simulink model "EngineModel_scaled_15_7_2016_with_new_maps"  (R2021a)
settings: Solver=ode4  StartTime=0.0  StopTime=30  FixedStep=0.2  RelTol=1e-3  EnableMultiTasking=on
values from neighbouring files (symbols this model uses):
  Fanmap_2 = [1 1 1 1 1 1 1 1 1 1 275.724 325.4224 ... (330 elements, 10x3x11)]    [enginemaps2.mat]
  HPCompmap_2 = [1 1 1 1 1 1 1 1 1 1 32.390865 37.6623195 ... (330 elements, 10x3x11)]    [enginemaps2.mat]
  HPTurbinemap_2 = [0.24979968 0.24979968 0.24979968 0.24979968 0.24979968 0.24979968 0.24979968 0.24979968 0.24979968 0.24979968 0.004250667 0.005047667 ... (330 elements, 10x3x11)]    [enginemaps2.mat]
  LPCompmap_2 = [1 1 1 1 1 1 1 1 1 1 34.17260994 40.23277722 ... (330 elements, 10x3x11)]    [enginemaps2.mat]
  LPTurbinemap_2 = [0.665969797 0.665969797 0.665969797 0.665969797 0.665969797 0.665969797 0.665969797 0.665969797 0.00912 0.013173333 0.015706667 0.01672 ... (264 elements, 8x3x11)]    [enginemaps2.mat]
undefined symbols (not defined in the file or in its folder): Adiabatic_compression_fan, Adiabatic_compression_HPC, Adiabatic_compression_LPC, coldnozzle, compression_ram, cond_f2, D, datatables, hotnozzle, HPT1, if_Nth, if_Ntl, if_Z, LPT, performance1, thermo_combustor, turbo
libraries: dspmtrx3 x10, aerolibatmos2 x8, dspsigattribs x3, dspsolvers x2, dspfactors x1
(part 13 of 13)

== system EngineModel_scaled_15_7_2016_with_new_maps/Double spool TFE CF6-50 steady state modeling (BOING 747-200)/Error Due to Vs/Error Due To Dv6/LPT/enthalpy_MAPS/LPT map/LPT Map lookup Table (DH//T) ==
  corr speed Ntl : Inport
  TFtl : Inport  Port=2
  3D LPTurbinemap Lookup Table (DH/T) : Lookup_n-D  NumberOfTableDimensions=3  BreakpointsForDimension1=[461.059151,535.7395809,608.9086832,673.9999999,735.0784813,781.7211783,815.12673,850.3562978]  BreakpointsForDimension2=[1,2,3]  BreakpointsForDimension3=[0,0.1,0.2,0.3,0.4,0.5,0.6,0.7,0.8,0.9,1]  IndexSearchMethod=Linear search  Table=LPTurbinemap_2  InterpMethod=Cubic spline  ExtrapMethod=Cubic spline  OutDataTypeStr=double  RndMeth=Simplest
      settings: InputPortMap=u0,u1,u2
  Constant1 : Constant  Value=2
  Display : Display
  If condition Ztl : Subsystem
  if_Ntl : Subsystem
  LPT (DH/T)tl : Outport
  wires:
  corr speed Ntl/1 -> if_Ntl/2(Ntl)
  if_Ntl/1(Ztli) -> If condition Ztl/1(Ztli)
  If condition Ztl/1(Ztl) -> 3D LPTurbinemap Lookup Table (DH/T)/3
  TFtl/1 -> 3D LPTurbinemap Lookup Table (DH/T)/1, if_Ntl/1(TFtl)
  Constant1/1 -> 3D LPTurbinemap Lookup Table (DH/T)/2
  3D LPTurbinemap Lookup Table (DH/T)/1 -> Display/1, LPT (DH/T)tl/1

== system EngineModel_scaled_15_7_2016_with_new_maps/Double spool TFE CF6-50 steady state modeling (BOING 747-200)/Error Due to Vs/Error Due To Dv6/LPT/enthalpy_MAPS/LPT map/LPT Map lookup Table Efficency ==
  corr speed Ntl : Inport
  TFtl : Inport  Port=2
  3D LPTurbinemap Lookup Table Effienicy : Lookup_n-D  NumberOfTableDimensions=3  BreakpointsForDimension1=[461.059151,535.7395809,608.9086832,673.9999999,735.0784813,781.7211783,815.12673,850.3562978]  BreakpointsForDimension2=[1,2,3]  BreakpointsForDimension3=[0,0.1,0.2,0.3,0.4,0.5,0.6,0.7,0.8,0.9,1]  IndexSearchMethod=Linear search  Table=LPTurbinemap_2  InterpMethod=Cubic spline  ExtrapMethod=Cubic spline  OutDataTypeStr=double  RndMeth=Simplest
      settings: InputPortMap=u0,u1,u2
  Constant1 : Constant  Value=3
  Display : Display
  If condition Ztl : Subsystem
  if_Ntl : Subsystem
  HPT Ettatl : Outport
  wires:
  corr speed Ntl/1 -> if_Ntl/2(Ntl)
  if_Ntl/1(Ztli) -> If condition Ztl/1(Ztli)
  If condition Ztl/1(Ztl) -> 3D LPTurbinemap Lookup Table Effienicy/3
  TFtl/1 -> 3D LPTurbinemap Lookup Table Effienicy/1, if_Ntl/1(TFtl)
  Constant1/1 -> 3D LPTurbinemap Lookup Table Effienicy/2
  3D LPTurbinemap Lookup Table Effienicy/1 -> Display/1, HPT Ettatl/1

== system EngineModel_scaled_15_7_2016_with_new_maps/Double spool TFE CF6-50 steady state modeling (BOING 747-200)/Error Due to Vs/Error Due To Dv7/HPT/enthalpy_MAPS/HPT map/HPT Map lookup Table (DH//T) ==
  corr speed Nth : Inport
  TFth : Inport  Port=2
  3D HPTurbinemap Lookup Table (DH/T) : Lookup_n-D  NumberOfTableDimensions=3  BreakpointsForDimension1=[124.08776,134.47272,148.45488,152.05208,153.8194,155.1488,156.4,157.7294,159.27776,161.3266]  BreakpointsForDimension2=[1,2,3]  BreakpointsForDimension3=[0,0.1,0.2,0.3,0.4,0.5,0.6,0.7,0.8,0.9,1]  IndexSearchMethod=Linear search  Table=HPTurbinemap_2  InterpMethod=Cubic spline  ExtrapMethod=Cubic spline  OutDataTypeStr=double  RndMeth=Simplest
      settings: InputPortMap=u0,u1,u2
  Constant1 : Constant  Value=2
  Display : Display
  If condition Zth : Subsystem
  if_Nth : Subsystem
  HPT (DH/T)th : Outport
  wires:
  3D HPTurbinemap Lookup Table (DH/T)/1 -> HPT (DH/T)th/1, Display/1
  TFth/1 -> if_Nth/1(TFth), 3D HPTurbinemap Lookup Table (DH/T)/1
  Constant1/1 -> 3D HPTurbinemap Lookup Table (DH/T)/2
  If condition Zth/1(Zth) -> 3D HPTurbinemap Lookup Table (DH/T)/3
  if_Nth/1(Zthi) -> If condition Zth/1(Zthi)
  corr speed Nth/1 -> if_Nth/2(Nth)

== system EngineModel_scaled_15_7_2016_with_new_maps/Double spool TFE CF6-50 steady state modeling (BOING 747-200)/Error Due to Vs/Error Due To Dv7/HPT/enthalpy_MAPS/HPT map/HPT Map lookup Table Efficency ==
  corr speed Nth : Inport
  TFth : Inport  Port=2
  3D HPTurbinemap Lookup Table Efficency : Lookup_n-D  NumberOfTableDimensions=3  BreakpointsForDimension1=[124.08776,134.47272,148.45488,152.05208,153.8194,155.1488,156.4,157.7294,159.27776,161.3266]  BreakpointsForDimension2=[1,2,3]  BreakpointsForDimension3=[0,0.1,0.2,0.3,0.4,0.5,0.6,0.7,0.8,0.9,1]  IndexSearchMethod=Linear search  Table=HPTurbinemap_2  InterpMethod=Cubic spline  ExtrapMethod=Cubic spline  OutDataTypeStr=double  RndMeth=Simplest
      settings: InputPortMap=u0,u1,u2
  Constant1 : Constant  Value=3
  Display : Display
  Display1 : Display
  If condition Zf : Subsystem
  if_Nth : Subsystem
  HPT Ettath : Outport
  wires:
  3D HPTurbinemap Lookup Table Efficency/1 -> HPT Ettath/1, Display/1
  Constant1/1 -> 3D HPTurbinemap Lookup Table Efficency/2
  TFth/1 -> if_Nth/1(TFth), 3D HPTurbinemap Lookup Table Efficency/1
  if_Nth/1(Zthi) -> If condition Zf/1(Zthi)
  corr speed Nth/1 -> if_Nth/2(Nth)
  If condition Zf/1(Zth) -> Display1/1, 3D HPTurbinemap Lookup Table Efficency/3

== system EngineModel_scaled_15_7_2016_with_new_maps/Double spool TFE CF6-50 steady state modeling (BOING 747-200)/Error Due to Vs/Error Due To Dv7/LPT/enthalpy_MAPS/LPT map/LPT Map lookup Table (DH//T) ==
  corr speed Ntl : Inport
  TFtl : Inport  Port=2
  3D LPTurbinemap Lookup Table (DH/T) : Lookup_n-D  NumberOfTableDimensions=3  BreakpointsForDimension1=[461.059151,535.7395809,608.9086832,673.9999999,735.0784813,781.7211783,815.12673,850.3562978]  BreakpointsForDimension2=[1,2,3]  BreakpointsForDimension3=[0,0.1,0.2,0.3,0.4,0.5,0.6,0.7,0.8,0.9,1]  IndexSearchMethod=Linear search  Table=LPTurbinemap_2  InterpMethod=Cubic spline  ExtrapMethod=Cubic spline  OutDataTypeStr=double  RndMeth=Simplest
      settings: InputPortMap=u0,u1,u2
  Constant1 : Constant  Value=2
  Display : Display
  If condition Ztl : Subsystem
  if_Ntl : Subsystem
  LPT (DH/T)tl : Outport
  wires:
  3D LPTurbinemap Lookup Table (DH/T)/1 -> LPT (DH/T)tl/1, Display/1
  Constant1/1 -> 3D LPTurbinemap Lookup Table (DH/T)/2
  TFtl/1 -> if_Ntl/1(TFtl), 3D LPTurbinemap Lookup Table (DH/T)/1
  If condition Ztl/1(Ztl) -> 3D LPTurbinemap Lookup Table (DH/T)/3
  if_Ntl/1(Ztli) -> If condition Ztl/1(Ztli)
  corr speed Ntl/1 -> if_Ntl/2(Ntl)

== system EngineModel_scaled_15_7_2016_with_new_maps/Double spool TFE CF6-50 steady state modeling (BOING 747-200)/Error Due to Vs/Error Due To Dv7/LPT/enthalpy_MAPS/LPT map/LPT Map lookup Table Efficency ==
  corr speed Ntl : Inport
  TFtl : Inport  Port=2
  3D LPTurbinemap Lookup Table Effienicy : Lookup_n-D  NumberOfTableDimensions=3  BreakpointsForDimension1=[461.059151,535.7395809,608.9086832,673.9999999,735.0784813,781.7211783,815.12673,850.3562978]  BreakpointsForDimension2=[1,2,3]  BreakpointsForDimension3=[0,0.1,0.2,0.3,0.4,0.5,0.6,0.7,0.8,0.9,1]  IndexSearchMethod=Linear search  Table=LPTurbinemap_2  InterpMethod=Cubic spline  ExtrapMethod=Cubic spline  OutDataTypeStr=double  RndMeth=Simplest
      settings: InputPortMap=u0,u1,u2
  Constant1 : Constant  Value=3
  Display : Display
  If condition Ztl : Subsystem
  if_Ntl : Subsystem
  HPT Ettatl : Outport
  wires:
  3D LPTurbinemap Lookup Table Effienicy/1 -> HPT Ettatl/1, Display/1
  Constant1/1 -> 3D LPTurbinemap Lookup Table Effienicy/2
  TFtl/1 -> if_Ntl/1(TFtl), 3D LPTurbinemap Lookup Table Effienicy/1
  If condition Ztl/1(Ztl) -> 3D LPTurbinemap Lookup Table Effienicy/3
  if_Ntl/1(Ztli) -> If condition Ztl/1(Ztli)
  corr speed Ntl/1 -> if_Ntl/2(Ntl)

== system EngineModel_scaled_15_7_2016_with_new_maps/Double spool TFE CF6-50 steady state modeling (BOING 747-200)/Off- Design Module/HPT/enthalpy_MAPS/HPT map/HPT Map lookup Table (DH//T)/If condition Zth ==
  Zthi : Inport
  Demux : Demux  Outputs=1
      settings: DisplayOption=none
  Interpreted MATLAB Function : MATLABFcn  MATLABFcn=if_Z(u(1))  OutputDimensions=1
  Mux : Mux  Inputs=1
      settings: DisplayOption=signals
  Zth : Outport
  wires:
  Interpreted MATLAB Function/1 -> Demux/1
  Mux/1 -> Interpreted MATLAB Function/1
  Demux/1 -> Zth/1
  Zthi/1 -> Mux/1

== system EngineModel_scaled_15_7_2016_with_new_maps/Double spool TFE CF6-50 steady state modeling (BOING 747-200)/Off- Design Module/HPT/enthalpy_MAPS/HPT map/HPT Map lookup Table (DH//T)/if_Nth ==
  TFth : Inport
  Nth : Inport  Port=2
  Demux : Demux  Outputs=1
      settings: DisplayOption=none
  Interpreted MATLAB Function : MATLABFcn  MATLABFcn=if_Nth(u(1),u(2))  OutputDimensions=1
  Mux : Mux  Inputs=2
      settings: DisplayOption=signals
  Zthi : Outport
  wires:
  Interpreted MATLAB Function/1 -> Demux/1
  TFth/1 -> Mux/1
  Mux/1 -> Interpreted MATLAB Function/1
  Demux/1 -> Zthi/1
  Nth/1 -> Mux/2

== system EngineModel_scaled_15_7_2016_with_new_maps/Double spool TFE CF6-50 steady state modeling (BOING 747-200)/Off- Design Module/HPT/enthalpy_MAPS/HPT map/HPT Map lookup Table Efficency/If condition Zf ==
  Zthi : Inport
  Demux : Demux  Outputs=1
      settings: DisplayOption=none
  Interpreted MATLAB Function : MATLABFcn  MATLABFcn=if_Z(u(1))  OutputDimensions=1
  Mux : Mux  Inputs=1
      settings: DisplayOption=signals
  Zth : Outport
  wires:
  Interpreted MATLAB Function/1 -> Demux/1
  Mux/1 -> Interpreted MATLAB Function/1
  Demux/1 -> Zth/1
  Zthi/1 -> Mux/1

== system EngineModel_scaled_15_7_2016_with_new_maps/Double spool TFE CF6-50 steady state modeling (BOING 747-200)/Off- Design Module/HPT/enthalpy_MAPS/HPT map/HPT Map lookup Table Efficency/if_Nth ==
  TFth : Inport
  Nth : Inport  Port=2
  Demux : Demux  Outputs=1
      settings: DisplayOption=none
  Interpreted MATLAB Function : MATLABFcn  MATLABFcn=if_Nth(u(1),u(2))  OutputDimensions=1
  Mux : Mux  Inputs=2
      settings: DisplayOption=signals
  Zthi : Outport
  wires:
  Interpreted MATLAB Function/1 -> Demux/1
  TFth/1 -> Mux/1
  Mux/1 -> Interpreted MATLAB Function/1
  Demux/1 -> Zthi/1
  Nth/1 -> Mux/2

== system EngineModel_scaled_15_7_2016_with_new_maps/Double spool TFE CF6-50 steady state modeling (BOING 747-200)/Off- Design Module/LPT/enthalpy_MAPS/LPT map/LPT Map lookup Table (DH//T)/If condition Ztl ==
  Ztli : Inport
  Demux : Demux  Outputs=1
      settings: DisplayOption=none
  Interpreted MATLAB Function : MATLABFcn  MATLABFcn=if_Z(u(1))  OutputDimensions=1
  Mux : Mux  Inputs=1
      settings: DisplayOption=signals
  Ztl : Outport
  wires:
  Interpreted MATLAB Function/1 -> Demux/1
  Mux/1 -> Interpreted MATLAB Function/1
  Demux/1 -> Ztl/1
  Ztli/1 -> Mux/1

== system EngineModel_scaled_15_7_2016_with_new_maps/Double spool TFE CF6-50 steady state modeling (BOING 747-200)/Off- Design Module/LPT/enthalpy_MAPS/LPT map/LPT Map lookup Table (DH//T)/if_Ntl ==
  TFtl : Inport
  Ntl : Inport  Port=2
  Demux : Demux  Outputs=1
      settings: DisplayOption=none
  Interpreted MATLAB Function : MATLABFcn  MATLABFcn=if_Ntl(u(1),u(2))  OutputDimensions=1
  Mux : Mux  Inputs=2
      settings: DisplayOption=signals
  Ztli : Outport
  wires:
  Interpreted MATLAB Function/1 -> Demux/1
  TFtl/1 -> Mux/1
  Mux/1 -> Interpreted MATLAB Function/1
  Demux/1 -> Ztli/1
  Ntl/1 -> Mux/2

== system EngineModel_scaled_15_7_2016_with_new_maps/Double spool TFE CF6-50 steady state modeling (BOING 747-200)/Off- Design Module/LPT/enthalpy_MAPS/LPT map/LPT Map lookup Table Efficency/If condition Ztl ==
  Ztli : Inport
  Demux : Demux  Outputs=1
      settings: DisplayOption=none
  Interpreted MATLAB Function : MATLABFcn  MATLABFcn=if_Z(u(1))  OutputDimensions=1
  Mux : Mux  Inputs=1
      settings: DisplayOption=signals
  Ztl : Outport
  wires:
  Interpreted MATLAB Function/1 -> Demux/1
  Mux/1 -> Interpreted MATLAB Function/1
  Demux/1 -> Ztl/1
  Ztli/1 -> Mux/1

== system EngineModel_scaled_15_7_2016_with_new_maps/Double spool TFE CF6-50 steady state modeling (BOING 747-200)/Off- Design Module/LPT/enthalpy_MAPS/LPT map/LPT Map lookup Table Efficency/if_Ntl ==
  TFtl : Inport
  Ntl : Inport  Port=2
  Demux : Demux  Outputs=1
      settings: DisplayOption=none
  Interpreted MATLAB Function : MATLABFcn  MATLABFcn=if_Ntl(u(1),u(2))  OutputDimensions=1
  Mux : Mux  Inputs=2
      settings: DisplayOption=signals
  Ztli : Outport
  wires:
  Interpreted MATLAB Function/1 -> Demux/1
  TFtl/1 -> Mux/1
  Mux/1 -> Interpreted MATLAB Function/1
  Demux/1 -> Ztli/1
  Ntl/1 -> Mux/2

== system EngineModel_scaled_15_7_2016_with_new_maps/Double spool TFE CF6-50 steady state modeling (BOING 747-200)/Error Due to Vs/Error Due To Dv1/HPT/enthalpy_MAPS/HPT map/HPT Map lookup Table (DH//T)/If condition Zth ==
  Zthi : Inport
  Demux : Demux  Outputs=1
      settings: DisplayOption=none
  Interpreted MATLAB Function : MATLABFcn  MATLABFcn=if_Z(u(1))  OutputDimensions=1
  Mux : Mux  Inputs=1
      settings: DisplayOption=signals
  Zth : Outport
  wires:
  Interpreted MATLAB Function/1 -> Demux/1
  Mux/1 -> Interpreted MATLAB Function/1
  Demux/1 -> Zth/1
  Zthi/1 -> Mux/1

== system EngineModel_scaled_15_7_2016_with_new_maps/Double spool TFE CF6-50 steady state modeling (BOING 747-200)/Error Due to Vs/Error Due To Dv1/HPT/enthalpy_MAPS/HPT map/HPT Map lookup Table (DH//T)/if_Nth ==
  TFth : Inport
  Nth : Inport  Port=2
  Demux : Demux  Outputs=1
      settings: DisplayOption=none
  Interpreted MATLAB Function : MATLABFcn  MATLABFcn=if_Nth(u(1),u(2))  OutputDimensions=1
  Mux : Mux  Inputs=2
      settings: DisplayOption=signals
  Zthi : Outport
  wires:
  Interpreted MATLAB Function/1 -> Demux/1
  TFth/1 -> Mux/1
  Mux/1 -> Interpreted MATLAB Function/1
  Demux/1 -> Zthi/1
  Nth/1 -> Mux/2

== system EngineModel_scaled_15_7_2016_with_new_maps/Double spool TFE CF6-50 steady state modeling (BOING 747-200)/Error Due to Vs/Error Due To Dv1/HPT/enthalpy_MAPS/HPT map/HPT Map lookup Table Efficency/If condition Zf ==
  Zthi : Inport
  Demux : Demux  Outputs=1
      settings: DisplayOption=none
  Interpreted MATLAB Function : MATLABFcn  MATLABFcn=if_Z(u(1))  OutputDimensions=1
  Mux : Mux  Inputs=1
      settings: DisplayOption=signals
  Zth : Outport
  wires:
  Interpreted MATLAB Function/1 -> Demux/1
  Mux/1 -> Interpreted MATLAB Function/1
  Demux/1 -> Zth/1
  Zthi/1 -> Mux/1

== system EngineModel_scaled_15_7_2016_with_new_maps/Double spool TFE CF6-50 steady state modeling (BOING 747-200)/Error Due to Vs/Error Due To Dv1/HPT/enthalpy_MAPS/HPT map/HPT Map lookup Table Efficency/if_Nth ==
  TFth : Inport
  Nth : Inport  Port=2
  Demux : Demux  Outputs=1
      settings: DisplayOption=none
  Interpreted MATLAB Function : MATLABFcn  MATLABFcn=if_Nth(u(1),u(2))  OutputDimensions=1
  Mux : Mux  Inputs=2
      settings: DisplayOption=signals
  Zthi : Outport
  wires:
  Interpreted MATLAB Function/1 -> Demux/1
  TFth/1 -> Mux/1
  Mux/1 -> Interpreted MATLAB Function/1
  Demux/1 -> Zthi/1
  Nth/1 -> Mux/2

== system EngineModel_scaled_15_7_2016_with_new_maps/Double spool TFE CF6-50 steady state modeling (BOING 747-200)/Error Due to Vs/Error Due To Dv1/LPT/enthalpy_MAPS/LPT map/LPT Map lookup Table (DH//T)/If condition Ztl ==
  Ztli : Inport
  Demux : Demux  Outputs=1
      settings: DisplayOption=none
  Interpreted MATLAB Function : MATLABFcn  MATLABFcn=if_Z(u(1))  OutputDimensions=1
  Mux : Mux  Inputs=1
      settings: DisplayOption=signals
  Ztl : Outport
  wires:
  Interpreted MATLAB Function/1 -> Demux/1
  Mux/1 -> Interpreted MATLAB Function/1
  Demux/1 -> Ztl/1
  Ztli/1 -> Mux/1

== system EngineModel_scaled_15_7_2016_with_new_maps/Double spool TFE CF6-50 steady state modeling (BOING 747-200)/Error Due to Vs/Error Due To Dv1/LPT/enthalpy_MAPS/LPT map/LPT Map lookup Table (DH//T)/if_Ntl ==
  TFtl : Inport
  Ntl : Inport  Port=2
  Demux : Demux  Outputs=1
      settings: DisplayOption=none
  Interpreted MATLAB Function : MATLABFcn  MATLABFcn=if_Ntl(u(1),u(2))  OutputDimensions=1
  Mux : Mux  Inputs=2
      settings: DisplayOption=signals
  Ztli : Outport
  wires:
  Interpreted MATLAB Function/1 -> Demux/1
  TFtl/1 -> Mux/1
  Mux/1 -> Interpreted MATLAB Function/1
  Demux/1 -> Ztli/1
  Ntl/1 -> Mux/2

== system EngineModel_scaled_15_7_2016_with_new_maps/Double spool TFE CF6-50 steady state modeling (BOING 747-200)/Error Due to Vs/Error Due To Dv1/LPT/enthalpy_MAPS/LPT map/LPT Map lookup Table Efficency/If condition Ztl ==
  Ztli : Inport
  Demux : Demux  Outputs=1
      settings: DisplayOption=none
  Interpreted MATLAB Function : MATLABFcn  MATLABFcn=if_Z(u(1))  OutputDimensions=1
  Mux : Mux  Inputs=1
      settings: DisplayOption=signals
  Ztl : Outport
  wires:
  Interpreted MATLAB Function/1 -> Demux/1
  Mux/1 -> Interpreted MATLAB Function/1
  Demux/1 -> Ztl/1
  Ztli/1 -> Mux/1

== system EngineModel_scaled_15_7_2016_with_new_maps/Double spool TFE CF6-50 steady state modeling (BOING 747-200)/Error Due to Vs/Error Due To Dv1/LPT/enthalpy_MAPS/LPT map/LPT Map lookup Table Efficency/if_Ntl ==
  TFtl : Inport
  Ntl : Inport  Port=2
  Demux : Demux  Outputs=1
      settings: DisplayOption=none
  Interpreted MATLAB Function : MATLABFcn  MATLABFcn=if_Ntl(u(1),u(2))  OutputDimensions=1
  Mux : Mux  Inputs=2
      settings: DisplayOption=signals
  Ztli : Outport
  wires:
  Interpreted MATLAB Function/1 -> Demux/1
  TFtl/1 -> Mux/1
  Mux/1 -> Interpreted MATLAB Function/1
  Demux/1 -> Ztli/1
  Ntl/1 -> Mux/2

== system EngineModel_scaled_15_7_2016_with_new_maps/Double spool TFE CF6-50 steady state modeling (BOING 747-200)/Error Due to Vs/Error Due To Dv2/HPT/enthalpy_MAPS/HPT map/HPT Map lookup Table (DH//T)/If condition Zth ==
  Zthi : Inport
  Demux : Demux  Outputs=1
      settings: DisplayOption=none
  Interpreted MATLAB Function : MATLABFcn  MATLABFcn=if_Z(u(1))  OutputDimensions=1
  Mux : Mux  Inputs=1
      settings: DisplayOption=signals
  Zth : Outport
  wires:
  Zthi/1 -> Mux/1
  Demux/1 -> Zth/1
  Mux/1 -> Interpreted MATLAB Function/1
  Interpreted MATLAB Function/1 -> Demux/1

== system EngineModel_scaled_15_7_2016_with_new_maps/Double spool TFE CF6-50 steady state modeling (BOING 747-200)/Error Due to Vs/Error Due To Dv2/HPT/enthalpy_MAPS/HPT map/HPT Map lookup Table (DH//T)/if_Nth ==
  TFth : Inport
  Nth : Inport  Port=2
  Demux : Demux  Outputs=1
      settings: DisplayOption=none
  Interpreted MATLAB Function : MATLABFcn  MATLABFcn=if_Nth(u(1),u(2))  OutputDimensions=1
  Mux : Mux  Inputs=2
      settings: DisplayOption=signals
  Zthi : Outport
  wires:
  Nth/1 -> Mux/2
  Demux/1 -> Zthi/1
  Mux/1 -> Interpreted MATLAB Function/1
  TFth/1 -> Mux/1
  Interpreted MATLAB Function/1 -> Demux/1

== system EngineModel_scaled_15_7_2016_with_new_maps/Double spool TFE CF6-50 steady state modeling (BOING 747-200)/Error Due to Vs/Error Due To Dv2/HPT/enthalpy_MAPS/HPT map/HPT Map lookup Table Efficency/If condition Zf ==
  Zthi : Inport
  Demux : Demux  Outputs=1
      settings: DisplayOption=none
  Interpreted MATLAB Function : MATLABFcn  MATLABFcn=if_Z(u(1))  OutputDimensions=1
  Mux : Mux  Inputs=1
      settings: DisplayOption=signals
  Zth : Outport
  wires:
  Zthi/1 -> Mux/1
  Demux/1 -> Zth/1
  Mux/1 -> Interpreted MATLAB Function/1
  Interpreted MATLAB Function/1 -> Demux/1

== system EngineModel_scaled_15_7_2016_with_new_maps/Double spool TFE CF6-50 steady state modeling (BOING 747-200)/Error Due to Vs/Error Due To Dv2/HPT/enthalpy_MAPS/HPT map/HPT Map lookup Table Efficency/if_Nth ==
  TFth : Inport
  Nth : Inport  Port=2
  Demux : Demux  Outputs=1
      settings: DisplayOption=none
  Interpreted MATLAB Function : MATLABFcn  MATLABFcn=if_Nth(u(1),u(2))  OutputDimensions=1
  Mux : Mux  Inputs=2
      settings: DisplayOption=signals
  Zthi : Outport
  wires:
  Nth/1 -> Mux/2
  Demux/1 -> Zthi/1
  Mux/1 -> Interpreted MATLAB Function/1
  TFth/1 -> Mux/1
  Interpreted MATLAB Function/1 -> Demux/1

== system EngineModel_scaled_15_7_2016_with_new_maps/Double spool TFE CF6-50 steady state modeling (BOING 747-200)/Error Due to Vs/Error Due To Dv2/LPT/enthalpy_MAPS/LPT map/LPT Map lookup Table (DH//T)/If condition Ztl ==
  Ztli : Inport
  Demux : Demux  Outputs=1
      settings: DisplayOption=none
  Interpreted MATLAB Function : MATLABFcn  MATLABFcn=if_Z(u(1))  OutputDimensions=1
  Mux : Mux  Inputs=1
      settings: DisplayOption=signals
  Ztl : Outport
  wires:
  Ztli/1 -> Mux/1
  Demux/1 -> Ztl/1
  Mux/1 -> Interpreted MATLAB Function/1
  Interpreted MATLAB Function/1 -> Demux/1

== system EngineModel_scaled_15_7_2016_with_new_maps/Double spool TFE CF6-50 steady state modeling (BOING 747-200)/Error Due to Vs/Error Due To Dv2/LPT/enthalpy_MAPS/LPT map/LPT Map lookup Table (DH//T)/if_Ntl ==
  TFtl : Inport
  Ntl : Inport  Port=2
  Demux : Demux  Outputs=1
      settings: DisplayOption=none
  Interpreted MATLAB Function : MATLABFcn  MATLABFcn=if_Ntl(u(1),u(2))  OutputDimensions=1
  Mux : Mux  Inputs=2
      settings: DisplayOption=signals
  Ztli : Outport
  wires:
  Ntl/1 -> Mux/2
  Demux/1 -> Ztli/1
  Mux/1 -> Interpreted MATLAB Function/1
  TFtl/1 -> Mux/1
  Interpreted MATLAB Function/1 -> Demux/1

== system EngineModel_scaled_15_7_2016_with_new_maps/Double spool TFE CF6-50 steady state modeling (BOING 747-200)/Error Due to Vs/Error Due To Dv2/LPT/enthalpy_MAPS/LPT map/LPT Map lookup Table Efficency/If condition Ztl ==
  Ztli : Inport
  Demux : Demux  Outputs=1
      settings: DisplayOption=none
  Interpreted MATLAB Function : MATLABFcn  MATLABFcn=if_Z(u(1))  OutputDimensions=1
  Mux : Mux  Inputs=1
      settings: DisplayOption=signals
  Ztl : Outport
  wires:
  Ztli/1 -> Mux/1
  Demux/1 -> Ztl/1
  Mux/1 -> Interpreted MATLAB Function/1
  Interpreted MATLAB Function/1 -> Demux/1

== system EngineModel_scaled_15_7_2016_with_new_maps/Double spool TFE CF6-50 steady state modeling (BOING 747-200)/Error Due to Vs/Error Due To Dv2/LPT/enthalpy_MAPS/LPT map/LPT Map lookup Table Efficency/if_Ntl ==
  TFtl : Inport
  Ntl : Inport  Port=2
  Demux : Demux  Outputs=1
      settings: DisplayOption=none
  Interpreted MATLAB Function : MATLABFcn  MATLABFcn=if_Ntl(u(1),u(2))  OutputDimensions=1
  Mux : Mux  Inputs=2
      settings: DisplayOption=signals
  Ztli : Outport
  wires:
  Ntl/1 -> Mux/2
  Demux/1 -> Ztli/1
  Mux/1 -> Interpreted MATLAB Function/1
  TFtl/1 -> Mux/1
  Interpreted MATLAB Function/1 -> Demux/1

== system EngineModel_scaled_15_7_2016_with_new_maps/Double spool TFE CF6-50 steady state modeling (BOING 747-200)/Error Due to Vs/Error Due To Dv3/HPT/enthalpy_MAPS/HPT map/HPT Map lookup Table (DH//T)/If condition Zth ==
  Zthi : Inport
  Demux : Demux  Outputs=1
      settings: DisplayOption=none
  Interpreted MATLAB Function : MATLABFcn  MATLABFcn=if_Z(u(1))  OutputDimensions=1
  Mux : Mux  Inputs=1
      settings: DisplayOption=signals
  Zth : Outport
  wires:
  Interpreted MATLAB Function/1 -> Demux/1
  Mux/1 -> Interpreted MATLAB Function/1
  Demux/1 -> Zth/1
  Zthi/1 -> Mux/1

== system EngineModel_scaled_15_7_2016_with_new_maps/Double spool TFE CF6-50 steady state modeling (BOING 747-200)/Error Due to Vs/Error Due To Dv3/HPT/enthalpy_MAPS/HPT map/HPT Map lookup Table (DH//T)/if_Nth ==
  TFth : Inport
  Nth : Inport  Port=2
  Demux : Demux  Outputs=1
      settings: DisplayOption=none
  Interpreted MATLAB Function : MATLABFcn  MATLABFcn=if_Nth(u(1),u(2))  OutputDimensions=1
  Mux : Mux  Inputs=2
      settings: DisplayOption=signals
  Zthi : Outport
  wires:
  Interpreted MATLAB Function/1 -> Demux/1
  TFth/1 -> Mux/1
  Mux/1 -> Interpreted MATLAB Function/1
  Demux/1 -> Zthi/1
  Nth/1 -> Mux/2

== system EngineModel_scaled_15_7_2016_with_new_maps/Double spool TFE CF6-50 steady state modeling (BOING 747-200)/Error Due to Vs/Error Due To Dv3/HPT/enthalpy_MAPS/HPT map/HPT Map lookup Table Efficency/If condition Zf ==
  Zthi : Inport
  Demux : Demux  Outputs=1
      settings: DisplayOption=none
  Interpreted MATLAB Function : MATLABFcn  MATLABFcn=if_Z(u(1))  OutputDimensions=1
  Mux : Mux  Inputs=1
      settings: DisplayOption=signals
  Zth : Outport
  wires:
  Interpreted MATLAB Function/1 -> Demux/1
  Mux/1 -> Interpreted MATLAB Function/1
  Demux/1 -> Zth/1
  Zthi/1 -> Mux/1

== system EngineModel_scaled_15_7_2016_with_new_maps/Double spool TFE CF6-50 steady state modeling (BOING 747-200)/Error Due to Vs/Error Due To Dv3/HPT/enthalpy_MAPS/HPT map/HPT Map lookup Table Efficency/if_Nth ==
  TFth : Inport
  Nth : Inport  Port=2
  Demux : Demux  Outputs=1
      settings: DisplayOption=none
  Interpreted MATLAB Function : MATLABFcn  MATLABFcn=if_Nth(u(1),u(2))  OutputDimensions=1
  Mux : Mux  Inputs=2
      settings: DisplayOption=signals
  Zthi : Outport
  wires:
  Interpreted MATLAB Function/1 -> Demux/1
  TFth/1 -> Mux/1
  Mux/1 -> Interpreted MATLAB Function/1
  Demux/1 -> Zthi/1
  Nth/1 -> Mux/2

== system EngineModel_scaled_15_7_2016_with_new_maps/Double spool TFE CF6-50 steady state modeling (BOING 747-200)/Error Due to Vs/Error Due To Dv3/LPT/enthalpy_MAPS/LPT map/LPT Map lookup Table (DH//T)/If condition Ztl ==
  Ztli : Inport
  Demux : Demux  Outputs=1
      settings: DisplayOption=none
  Interpreted MATLAB Function : MATLABFcn  MATLABFcn=if_Z(u(1))  OutputDimensions=1
  Mux : Mux  Inputs=1
      settings: DisplayOption=signals
  Ztl : Outport
  wires:
  Interpreted MATLAB Function/1 -> Demux/1
  Mux/1 -> Interpreted MATLAB Function/1
  Demux/1 -> Ztl/1
  Ztli/1 -> Mux/1

== system EngineModel_scaled_15_7_2016_with_new_maps/Double spool TFE CF6-50 steady state modeling (BOING 747-200)/Error Due to Vs/Error Due To Dv3/LPT/enthalpy_MAPS/LPT map/LPT Map lookup Table (DH//T)/if_Ntl ==
  TFtl : Inport
  Ntl : Inport  Port=2
  Demux : Demux  Outputs=1
      settings: DisplayOption=none
  Interpreted MATLAB Function : MATLABFcn  MATLABFcn=if_Ntl(u(1),u(2))  OutputDimensions=1
  Mux : Mux  Inputs=2
      settings: DisplayOption=signals
  Ztli : Outport
  wires:
  Interpreted MATLAB Function/1 -> Demux/1
  TFtl/1 -> Mux/1
  Mux/1 -> Interpreted MATLAB Function/1
  Demux/1 -> Ztli/1
  Ntl/1 -> Mux/2

== system EngineModel_scaled_15_7_2016_with_new_maps/Double spool TFE CF6-50 steady state modeling (BOING 747-200)/Error Due to Vs/Error Due To Dv3/LPT/enthalpy_MAPS/LPT map/LPT Map lookup Table Efficency/If condition Ztl ==
  Ztli : Inport
  Demux : Demux  Outputs=1
      settings: DisplayOption=none
  Interpreted MATLAB Function : MATLABFcn  MATLABFcn=if_Z(u(1))  OutputDimensions=1
  Mux : Mux  Inputs=1
      settings: DisplayOption=signals
  Ztl : Outport
  wires:
  Interpreted MATLAB Function/1 -> Demux/1
  Mux/1 -> Interpreted MATLAB Function/1
  Demux/1 -> Ztl/1
  Ztli/1 -> Mux/1

== system EngineModel_scaled_15_7_2016_with_new_maps/Double spool TFE CF6-50 steady state modeling (BOING 747-200)/Error Due to Vs/Error Due To Dv3/LPT/enthalpy_MAPS/LPT map/LPT Map lookup Table Efficency/if_Ntl ==
  TFtl : Inport
  Ntl : Inport  Port=2
  Demux : Demux  Outputs=1
      settings: DisplayOption=none
  Interpreted MATLAB Function : MATLABFcn  MATLABFcn=if_Ntl(u(1),u(2))  OutputDimensions=1
  Mux : Mux  Inputs=2
      settings: DisplayOption=signals
  Ztli : Outport
  wires:
  Interpreted MATLAB Function/1 -> Demux/1
  TFtl/1 -> Mux/1
  Mux/1 -> Interpreted MATLAB Function/1
  Demux/1 -> Ztli/1
  Ntl/1 -> Mux/2

== system EngineModel_scaled_15_7_2016_with_new_maps/Double spool TFE CF6-50 steady state modeling (BOING 747-200)/Error Due to Vs/Error Due To Dv4/HPT/enthalpy_MAPS/HPT map/HPT Map lookup Table (DH//T)/If condition Zth ==
  Zthi : Inport
  Demux : Demux  Outputs=1
      settings: DisplayOption=none
  Interpreted MATLAB Function : MATLABFcn  MATLABFcn=if_Z(u(1))  OutputDimensions=1
  Mux : Mux  Inputs=1
      settings: DisplayOption=signals
  Zth : Outport
  wires:
  Zthi/1 -> Mux/1
  Demux/1 -> Zth/1
  Mux/1 -> Interpreted MATLAB Function/1
  Interpreted MATLAB Function/1 -> Demux/1

== system EngineModel_scaled_15_7_2016_with_new_maps/Double spool TFE CF6-50 steady state modeling (BOING 747-200)/Error Due to Vs/Error Due To Dv4/HPT/enthalpy_MAPS/HPT map/HPT Map lookup Table (DH//T)/if_Nth ==
  TFth : Inport
  Nth : Inport  Port=2
  Demux : Demux  Outputs=1
      settings: DisplayOption=none
  Interpreted MATLAB Function : MATLABFcn  MATLABFcn=if_Nth(u(1),u(2))  OutputDimensions=1
  Mux : Mux  Inputs=2
      settings: DisplayOption=signals
  Zthi : Outport
  wires:
  Nth/1 -> Mux/2
  Demux/1 -> Zthi/1
  Mux/1 -> Interpreted MATLAB Function/1
  TFth/1 -> Mux/1
  Interpreted MATLAB Function/1 -> Demux/1

== system EngineModel_scaled_15_7_2016_with_new_maps/Double spool TFE CF6-50 steady state modeling (BOING 747-200)/Error Due to Vs/Error Due To Dv4/HPT/enthalpy_MAPS/HPT map/HPT Map lookup Table Efficency/If condition Zf ==
  Zthi : Inport
  Demux : Demux  Outputs=1
      settings: DisplayOption=none
  Interpreted MATLAB Function : MATLABFcn  MATLABFcn=if_Z(u(1))  OutputDimensions=1
  Mux : Mux  Inputs=1
      settings: DisplayOption=signals
  Zth : Outport
  wires:
  Zthi/1 -> Mux/1
  Demux/1 -> Zth/1
  Mux/1 -> Interpreted MATLAB Function/1
  Interpreted MATLAB Function/1 -> Demux/1

== system EngineModel_scaled_15_7_2016_with_new_maps/Double spool TFE CF6-50 steady state modeling (BOING 747-200)/Error Due to Vs/Error Due To Dv4/HPT/enthalpy_MAPS/HPT map/HPT Map lookup Table Efficency/if_Nth ==
  TFth : Inport
  Nth : Inport  Port=2
  Demux : Demux  Outputs=1
      settings: DisplayOption=none
  Interpreted MATLAB Function : MATLABFcn  MATLABFcn=if_Nth(u(1),u(2))  OutputDimensions=1
  Mux : Mux  Inputs=2
      settings: DisplayOption=signals
  Zthi : Outport
  wires:
  Nth/1 -> Mux/2
  Demux/1 -> Zthi/1
  Mux/1 -> Interpreted MATLAB Function/1
  TFth/1 -> Mux/1
  Interpreted MATLAB Function/1 -> Demux/1

== system EngineModel_scaled_15_7_2016_with_new_maps/Double spool TFE CF6-50 steady state modeling (BOING 747-200)/Error Due to Vs/Error Due To Dv4/LPT/enthalpy_MAPS/LPT map/LPT Map lookup Table (DH//T)/If condition Ztl ==
  Ztli : Inport
  Demux : Demux  Outputs=1
      settings: DisplayOption=none
  Interpreted MATLAB Function : MATLABFcn  MATLABFcn=if_Z(u(1))  OutputDimensions=1
  Mux : Mux  Inputs=1
      settings: DisplayOption=signals
  Ztl : Outport
  wires:
  Ztli/1 -> Mux/1
  Demux/1 -> Ztl/1
  Mux/1 -> Interpreted MATLAB Function/1
  Interpreted MATLAB Function/1 -> Demux/1

== system EngineModel_scaled_15_7_2016_with_new_maps/Double spool TFE CF6-50 steady state modeling (BOING 747-200)/Error Due to Vs/Error Due To Dv4/LPT/enthalpy_MAPS/LPT map/LPT Map lookup Table (DH//T)/if_Ntl ==
  TFtl : Inport
  Ntl : Inport  Port=2
  Demux : Demux  Outputs=1
      settings: DisplayOption=none
  Interpreted MATLAB Function : MATLABFcn  MATLABFcn=if_Ntl(u(1),u(2))  OutputDimensions=1
  Mux : Mux  Inputs=2
      settings: DisplayOption=signals
  Ztli : Outport
  wires:
  Ntl/1 -> Mux/2
  Demux/1 -> Ztli/1
  Mux/1 -> Interpreted MATLAB Function/1
  TFtl/1 -> Mux/1
  Interpreted MATLAB Function/1 -> Demux/1

== system EngineModel_scaled_15_7_2016_with_new_maps/Double spool TFE CF6-50 steady state modeling (BOING 747-200)/Error Due to Vs/Error Due To Dv4/LPT/enthalpy_MAPS/LPT map/LPT Map lookup Table Efficency/If condition Ztl ==
  Ztli : Inport
  Demux : Demux  Outputs=1
      settings: DisplayOption=none
  Interpreted MATLAB Function : MATLABFcn  MATLABFcn=if_Z(u(1))  OutputDimensions=1
  Mux : Mux  Inputs=1
      settings: DisplayOption=signals
  Ztl : Outport
  wires:
  Ztli/1 -> Mux/1
  Demux/1 -> Ztl/1
  Mux/1 -> Interpreted MATLAB Function/1
  Interpreted MATLAB Function/1 -> Demux/1

== system EngineModel_scaled_15_7_2016_with_new_maps/Double spool TFE CF6-50 steady state modeling (BOING 747-200)/Error Due to Vs/Error Due To Dv4/LPT/enthalpy_MAPS/LPT map/LPT Map lookup Table Efficency/if_Ntl ==
  TFtl : Inport
  Ntl : Inport  Port=2
  Demux : Demux  Outputs=1
      settings: DisplayOption=none
  Interpreted MATLAB Function : MATLABFcn  MATLABFcn=if_Ntl(u(1),u(2))  OutputDimensions=1
  Mux : Mux  Inputs=2
      settings: DisplayOption=signals
  Ztli : Outport
  wires:
  Ntl/1 -> Mux/2
  Demux/1 -> Ztli/1
  Mux/1 -> Interpreted MATLAB Function/1
  TFtl/1 -> Mux/1
  Interpreted MATLAB Function/1 -> Demux/1

== system EngineModel_scaled_15_7_2016_with_new_maps/Double spool TFE CF6-50 steady state modeling (BOING 747-200)/Error Due to Vs/Error Due To Dv5/HPT/enthalpy_MAPS/HPT map/HPT Map lookup Table (DH//T)/If condition Zth ==
  Zthi : Inport
  Demux : Demux  Outputs=1
      settings: DisplayOption=none
  Interpreted MATLAB Function : MATLABFcn  MATLABFcn=if_Z(u(1))  OutputDimensions=1
  Mux : Mux  Inputs=1
      settings: DisplayOption=signals
  Zth : Outport
  wires:
  Interpreted MATLAB Function/1 -> Demux/1
  Mux/1 -> Interpreted MATLAB Function/1
  Demux/1 -> Zth/1
  Zthi/1 -> Mux/1

== system EngineModel_scaled_15_7_2016_with_new_maps/Double spool TFE CF6-50 steady state modeling (BOING 747-200)/Error Due to Vs/Error Due To Dv5/HPT/enthalpy_MAPS/HPT map/HPT Map lookup Table (DH//T)/if_Nth ==
  TFth : Inport
  Nth : Inport  Port=2
  Demux : Demux  Outputs=1
      settings: DisplayOption=none
  Interpreted MATLAB Function : MATLABFcn  MATLABFcn=if_Nth(u(1),u(2))  OutputDimensions=1
  Mux : Mux  Inputs=2
      settings: DisplayOption=signals
  Zthi : Outport
  wires:
  Interpreted MATLAB Function/1 -> Demux/1
  TFth/1 -> Mux/1
  Mux/1 -> Interpreted MATLAB Function/1
  Demux/1 -> Zthi/1
  Nth/1 -> Mux/2

== system EngineModel_scaled_15_7_2016_with_new_maps/Double spool TFE CF6-50 steady state modeling (BOING 747-200)/Error Due to Vs/Error Due To Dv5/HPT/enthalpy_MAPS/HPT map/HPT Map lookup Table Efficency/If condition Zf ==
  Zthi : Inport
  Demux : Demux  Outputs=1
      settings: DisplayOption=none
  Interpreted MATLAB Function : MATLABFcn  MATLABFcn=if_Z(u(1))  OutputDimensions=1
  Mux : Mux  Inputs=1
      settings: DisplayOption=signals
  Zth : Outport
  wires:
  Interpreted MATLAB Function/1 -> Demux/1
  Mux/1 -> Interpreted MATLAB Function/1
  Demux/1 -> Zth/1
  Zthi/1 -> Mux/1

== system EngineModel_scaled_15_7_2016_with_new_maps/Double spool TFE CF6-50 steady state modeling (BOING 747-200)/Error Due to Vs/Error Due To Dv5/HPT/enthalpy_MAPS/HPT map/HPT Map lookup Table Efficency/if_Nth ==
  TFth : Inport
  Nth : Inport  Port=2
  Demux : Demux  Outputs=1
      settings: DisplayOption=none
  Interpreted MATLAB Function : MATLABFcn  MATLABFcn=if_Nth(u(1),u(2))  OutputDimensions=1
  Mux : Mux  Inputs=2
      settings: DisplayOption=signals
  Zthi : Outport
  wires:
  Interpreted MATLAB Function/1 -> Demux/1
  TFth/1 -> Mux/1
  Mux/1 -> Interpreted MATLAB Function/1
  Demux/1 -> Zthi/1
  Nth/1 -> Mux/2

== system EngineModel_scaled_15_7_2016_with_new_maps/Double spool TFE CF6-50 steady state modeling (BOING 747-200)/Error Due to Vs/Error Due To Dv5/LPT/enthalpy_MAPS/LPT map/LPT Map lookup Table (DH//T)/If condition Ztl ==
  Ztli : Inport
  Demux : Demux  Outputs=1
      settings: DisplayOption=none
  Interpreted MATLAB Function : MATLABFcn  MATLABFcn=if_Z(u(1))  OutputDimensions=1
  Mux : Mux  Inputs=1
      settings: DisplayOption=signals
  Ztl : Outport
  wires:
  Interpreted MATLAB Function/1 -> Demux/1
  Mux/1 -> Interpreted MATLAB Function/1
  Demux/1 -> Ztl/1
  Ztli/1 -> Mux/1

== system EngineModel_scaled_15_7_2016_with_new_maps/Double spool TFE CF6-50 steady state modeling (BOING 747-200)/Error Due to Vs/Error Due To Dv5/LPT/enthalpy_MAPS/LPT map/LPT Map lookup Table (DH//T)/if_Ntl ==
  TFtl : Inport
  Ntl : Inport  Port=2
  Demux : Demux  Outputs=1
      settings: DisplayOption=none
  Interpreted MATLAB Function : MATLABFcn  MATLABFcn=if_Ntl(u(1),u(2))  OutputDimensions=1
  Mux : Mux  Inputs=2
      settings: DisplayOption=signals
  Ztli : Outport
  wires:
  Interpreted MATLAB Function/1 -> Demux/1
  TFtl/1 -> Mux/1
  Mux/1 -> Interpreted MATLAB Function/1
  Demux/1 -> Ztli/1
  Ntl/1 -> Mux/2

== system EngineModel_scaled_15_7_2016_with_new_maps/Double spool TFE CF6-50 steady state modeling (BOING 747-200)/Error Due to Vs/Error Due To Dv5/LPT/enthalpy_MAPS/LPT map/LPT Map lookup Table Efficency/If condition Ztl ==
  Ztli : Inport
  Demux : Demux  Outputs=1
      settings: DisplayOption=none
  Interpreted MATLAB Function : MATLABFcn  MATLABFcn=if_Z(u(1))  OutputDimensions=1
  Mux : Mux  Inputs=1
      settings: DisplayOption=signals
  Ztl : Outport
  wires:
  Interpreted MATLAB Function/1 -> Demux/1
  Mux/1 -> Interpreted MATLAB Function/1
  Demux/1 -> Ztl/1
  Ztli/1 -> Mux/1

== system EngineModel_scaled_15_7_2016_with_new_maps/Double spool TFE CF6-50 steady state modeling (BOING 747-200)/Error Due to Vs/Error Due To Dv5/LPT/enthalpy_MAPS/LPT map/LPT Map lookup Table Efficency/if_Ntl ==
  TFtl : Inport
  Ntl : Inport  Port=2
  Demux : Demux  Outputs=1
      settings: DisplayOption=none
  Interpreted MATLAB Function : MATLABFcn  MATLABFcn=if_Ntl(u(1),u(2))  OutputDimensions=1
  Mux : Mux  Inputs=2
      settings: DisplayOption=signals
  Ztli : Outport
  wires:
  Interpreted MATLAB Function/1 -> Demux/1
  TFtl/1 -> Mux/1
  Mux/1 -> Interpreted MATLAB Function/1
  Demux/1 -> Ztli/1
  Ntl/1 -> Mux/2

== system EngineModel_scaled_15_7_2016_with_new_maps/Double spool TFE CF6-50 steady state modeling (BOING 747-200)/Error Due to Vs/Error Due To Dv6/HPT/enthalpy_MAPS/HPT map/HPT Map lookup Table (DH//T)/If condition Zth ==
  Zthi : Inport
  Demux : Demux  Outputs=1
      settings: DisplayOption=none
  Interpreted MATLAB Function : MATLABFcn  MATLABFcn=if_Z(u(1))  OutputDimensions=1
  Mux : Mux  Inputs=1
      settings: DisplayOption=signals
  Zth : Outport
  wires:
  Zthi/1 -> Mux/1
  Demux/1 -> Zth/1
  Mux/1 -> Interpreted MATLAB Function/1
  Interpreted MATLAB Function/1 -> Demux/1

== system EngineModel_scaled_15_7_2016_with_new_maps/Double spool TFE CF6-50 steady state modeling (BOING 747-200)/Error Due to Vs/Error Due To Dv6/HPT/enthalpy_MAPS/HPT map/HPT Map lookup Table (DH//T)/if_Nth ==
  TFth : Inport
  Nth : Inport  Port=2
  Demux : Demux  Outputs=1
      settings: DisplayOption=none
  Interpreted MATLAB Function : MATLABFcn  MATLABFcn=if_Nth(u(1),u(2))  OutputDimensions=1
  Mux : Mux  Inputs=2
      settings: DisplayOption=signals
  Zthi : Outport
  wires:
  Nth/1 -> Mux/2
  Demux/1 -> Zthi/1
  Mux/1 -> Interpreted MATLAB Function/1
  TFth/1 -> Mux/1
  Interpreted MATLAB Function/1 -> Demux/1

== system EngineModel_scaled_15_7_2016_with_new_maps/Double spool TFE CF6-50 steady state modeling (BOING 747-200)/Error Due to Vs/Error Due To Dv6/HPT/enthalpy_MAPS/HPT map/HPT Map lookup Table Efficency/If condition Zf ==
  Zthi : Inport
  Demux : Demux  Outputs=1
      settings: DisplayOption=none
  Interpreted MATLAB Function : MATLABFcn  MATLABFcn=if_Z(u(1))  OutputDimensions=1
  Mux : Mux  Inputs=1
      settings: DisplayOption=signals
  Zth : Outport
  wires:
  Zthi/1 -> Mux/1
  Demux/1 -> Zth/1
  Mux/1 -> Interpreted MATLAB Function/1
  Interpreted MATLAB Function/1 -> Demux/1

== system EngineModel_scaled_15_7_2016_with_new_maps/Double spool TFE CF6-50 steady state modeling (BOING 747-200)/Error Due to Vs/Error Due To Dv6/HPT/enthalpy_MAPS/HPT map/HPT Map lookup Table Efficency/if_Nth ==
  TFth : Inport
  Nth : Inport  Port=2
  Demux : Demux  Outputs=1
      settings: DisplayOption=none
  Interpreted MATLAB Function : MATLABFcn  MATLABFcn=if_Nth(u(1),u(2))  OutputDimensions=1
  Mux : Mux  Inputs=2
      settings: DisplayOption=signals
  Zthi : Outport
  wires:
  Nth/1 -> Mux/2
  Demux/1 -> Zthi/1
  Mux/1 -> Interpreted MATLAB Function/1
  TFth/1 -> Mux/1
  Interpreted MATLAB Function/1 -> Demux/1

== system EngineModel_scaled_15_7_2016_with_new_maps/Double spool TFE CF6-50 steady state modeling (BOING 747-200)/Error Due to Vs/Error Due To Dv6/LPT/enthalpy_MAPS/LPT map/LPT Map lookup Table (DH//T)/If condition Ztl ==
  Ztli : Inport
  Demux : Demux  Outputs=1
      settings: DisplayOption=none
  Interpreted MATLAB Function : MATLABFcn  MATLABFcn=if_Z(u(1))  OutputDimensions=1
  Mux : Mux  Inputs=1
      settings: DisplayOption=signals
  Ztl : Outport
  wires:
  Ztli/1 -> Mux/1
  Demux/1 -> Ztl/1
  Mux/1 -> Interpreted MATLAB Function/1
  Interpreted MATLAB Function/1 -> Demux/1

== system EngineModel_scaled_15_7_2016_with_new_maps/Double spool TFE CF6-50 steady state modeling (BOING 747-200)/Error Due to Vs/Error Due To Dv6/LPT/enthalpy_MAPS/LPT map/LPT Map lookup Table (DH//T)/if_Ntl ==
  TFtl : Inport
  Ntl : Inport  Port=2
  Demux : Demux  Outputs=1
      settings: DisplayOption=none
  Interpreted MATLAB Function : MATLABFcn  MATLABFcn=if_Ntl(u(1),u(2))  OutputDimensions=1
  Mux : Mux  Inputs=2
      settings: DisplayOption=signals
  Ztli : Outport
  wires:
  Ntl/1 -> Mux/2
  Demux/1 -> Ztli/1
  Mux/1 -> Interpreted MATLAB Function/1
  TFtl/1 -> Mux/1
  Interpreted MATLAB Function/1 -> Demux/1

== system EngineModel_scaled_15_7_2016_with_new_maps/Double spool TFE CF6-50 steady state modeling (BOING 747-200)/Error Due to Vs/Error Due To Dv6/LPT/enthalpy_MAPS/LPT map/LPT Map lookup Table Efficency/If condition Ztl ==
  Ztli : Inport
  Demux : Demux  Outputs=1
      settings: DisplayOption=none
  Interpreted MATLAB Function : MATLABFcn  MATLABFcn=if_Z(u(1))  OutputDimensions=1
  Mux : Mux  Inputs=1
      settings: DisplayOption=signals
  Ztl : Outport
  wires:
  Ztli/1 -> Mux/1
  Demux/1 -> Ztl/1
  Mux/1 -> Interpreted MATLAB Function/1
  Interpreted MATLAB Function/1 -> Demux/1

== system EngineModel_scaled_15_7_2016_with_new_maps/Double spool TFE CF6-50 steady state modeling (BOING 747-200)/Error Due to Vs/Error Due To Dv6/LPT/enthalpy_MAPS/LPT map/LPT Map lookup Table Efficency/if_Ntl ==
  TFtl : Inport
  Ntl : Inport  Port=2
  Demux : Demux  Outputs=1
      settings: DisplayOption=none
  Interpreted MATLAB Function : MATLABFcn  MATLABFcn=if_Ntl(u(1),u(2))  OutputDimensions=1
  Mux : Mux  Inputs=2
      settings: DisplayOption=signals
  Ztli : Outport
  wires:
  Ntl/1 -> Mux/2
  Demux/1 -> Ztli/1
  Mux/1 -> Interpreted MATLAB Function/1
  TFtl/1 -> Mux/1
  Interpreted MATLAB Function/1 -> Demux/1

== system EngineModel_scaled_15_7_2016_with_new_maps/Double spool TFE CF6-50 steady state modeling (BOING 747-200)/Error Due to Vs/Error Due To Dv7/HPT/enthalpy_MAPS/HPT map/HPT Map lookup Table (DH//T)/If condition Zth ==
  Zthi : Inport
  Demux : Demux  Outputs=1
      settings: DisplayOption=none
  Interpreted MATLAB Function : MATLABFcn  MATLABFcn=if_Z(u(1))  OutputDimensions=1
  Mux : Mux  Inputs=1
      settings: DisplayOption=signals
  Zth : Outport
  wires:
  Interpreted MATLAB Function/1 -> Demux/1
  Mux/1 -> Interpreted MATLAB Function/1
  Demux/1 -> Zth/1
  Zthi/1 -> Mux/1

== system EngineModel_scaled_15_7_2016_with_new_maps/Double spool TFE CF6-50 steady state modeling (BOING 747-200)/Error Due to Vs/Error Due To Dv7/HPT/enthalpy_MAPS/HPT map/HPT Map lookup Table (DH//T)/if_Nth ==
  TFth : Inport
  Nth : Inport  Port=2
  Demux : Demux  Outputs=1
      settings: DisplayOption=none
  Interpreted MATLAB Function : MATLABFcn  MATLABFcn=if_Nth(u(1),u(2))  OutputDimensions=1
  Mux : Mux  Inputs=2
      settings: DisplayOption=signals
  Zthi : Outport
  wires:
  Interpreted MATLAB Function/1 -> Demux/1
  TFth/1 -> Mux/1
  Mux/1 -> Interpreted MATLAB Function/1
  Demux/1 -> Zthi/1
  Nth/1 -> Mux/2

== system EngineModel_scaled_15_7_2016_with_new_maps/Double spool TFE CF6-50 steady state modeling (BOING 747-200)/Error Due to Vs/Error Due To Dv7/HPT/enthalpy_MAPS/HPT map/HPT Map lookup Table Efficency/If condition Zf ==
  Zthi : Inport
  Demux : Demux  Outputs=1
      settings: DisplayOption=none
  Interpreted MATLAB Function : MATLABFcn  MATLABFcn=if_Z(u(1))  OutputDimensions=1
  Mux : Mux  Inputs=1
      settings: DisplayOption=signals
  Zth : Outport
  wires:
  Interpreted MATLAB Function/1 -> Demux/1
  Mux/1 -> Interpreted MATLAB Function/1
  Demux/1 -> Zth/1
  Zthi/1 -> Mux/1

== system EngineModel_scaled_15_7_2016_with_new_maps/Double spool TFE CF6-50 steady state modeling (BOING 747-200)/Error Due to Vs/Error Due To Dv7/HPT/enthalpy_MAPS/HPT map/HPT Map lookup Table Efficency/if_Nth ==
  TFth : Inport
  Nth : Inport  Port=2
  Demux : Demux  Outputs=1
      settings: DisplayOption=none
  Interpreted MATLAB Function : MATLABFcn  MATLABFcn=if_Nth(u(1),u(2))  OutputDimensions=1
  Mux : Mux  Inputs=2
      settings: DisplayOption=signals
  Zthi : Outport
  wires:
  Interpreted MATLAB Function/1 -> Demux/1
  TFth/1 -> Mux/1
  Mux/1 -> Interpreted MATLAB Function/1
  Demux/1 -> Zthi/1
  Nth/1 -> Mux/2

== system EngineModel_scaled_15_7_2016_with_new_maps/Double spool TFE CF6-50 steady state modeling (BOING 747-200)/Error Due to Vs/Error Due To Dv7/LPT/enthalpy_MAPS/LPT map/LPT Map lookup Table (DH//T)/If condition Ztl ==
  Ztli : Inport
  Demux : Demux  Outputs=1
      settings: DisplayOption=none
  Interpreted MATLAB Function : MATLABFcn  MATLABFcn=if_Z(u(1))  OutputDimensions=1
  Mux : Mux  Inputs=1
      settings: DisplayOption=signals
  Ztl : Outport
  wires:
  Interpreted MATLAB Function/1 -> Demux/1
  Mux/1 -> Interpreted MATLAB Function/1
  Demux/1 -> Ztl/1
  Ztli/1 -> Mux/1

== system EngineModel_scaled_15_7_2016_with_new_maps/Double spool TFE CF6-50 steady state modeling (BOING 747-200)/Error Due to Vs/Error Due To Dv7/LPT/enthalpy_MAPS/LPT map/LPT Map lookup Table (DH//T)/if_Ntl ==
  TFtl : Inport
  Ntl : Inport  Port=2
  Demux : Demux  Outputs=1
      settings: DisplayOption=none
  Interpreted MATLAB Function : MATLABFcn  MATLABFcn=if_Ntl(u(1),u(2))  OutputDimensions=1
  Mux : Mux  Inputs=2
      settings: DisplayOption=signals
  Ztli : Outport
  wires:
  Interpreted MATLAB Function/1 -> Demux/1
  TFtl/1 -> Mux/1
  Mux/1 -> Interpreted MATLAB Function/1
  Demux/1 -> Ztli/1
  Ntl/1 -> Mux/2

== system EngineModel_scaled_15_7_2016_with_new_maps/Double spool TFE CF6-50 steady state modeling (BOING 747-200)/Error Due to Vs/Error Due To Dv7/LPT/enthalpy_MAPS/LPT map/LPT Map lookup Table Efficency/If condition Ztl ==
  Ztli : Inport
  Demux : Demux  Outputs=1
      settings: DisplayOption=none
  Interpreted MATLAB Function : MATLABFcn  MATLABFcn=if_Z(u(1))  OutputDimensions=1
  Mux : Mux  Inputs=1
      settings: DisplayOption=signals
  Ztl : Outport
  wires:
  Interpreted MATLAB Function/1 -> Demux/1
  Mux/1 -> Interpreted MATLAB Function/1
  Demux/1 -> Ztl/1
  Ztli/1 -> Mux/1

== system EngineModel_scaled_15_7_2016_with_new_maps/Double spool TFE CF6-50 steady state modeling (BOING 747-200)/Error Due to Vs/Error Due To Dv7/LPT/enthalpy_MAPS/LPT map/LPT Map lookup Table Efficency/if_Ntl ==
  TFtl : Inport
  Ntl : Inport  Port=2
  Demux : Demux  Outputs=1
      settings: DisplayOption=none
  Interpreted MATLAB Function : MATLABFcn  MATLABFcn=if_Ntl(u(1),u(2))  OutputDimensions=1
  Mux : Mux  Inputs=2
      settings: DisplayOption=signals
  Ztli : Outport
  wires:
  Interpreted MATLAB Function/1 -> Demux/1
  TFtl/1 -> Mux/1
  Mux/1 -> Interpreted MATLAB Function/1
  Demux/1 -> Ztli/1
  Ntl/1 -> Mux/2
